simulink model "test14"  (R2019b)
settings: Solver=VariableStepAuto  StartTime=0.0  StopTime=10.0  RelTol=1e-3
settings Model: Creator=maxim  LastModifiedBy=maxim

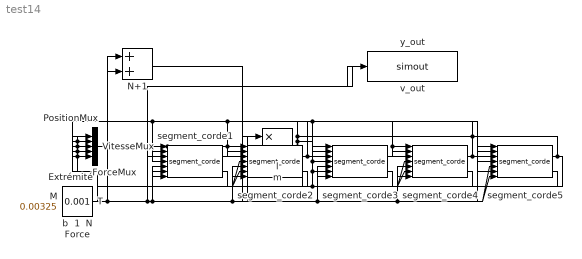
== system test14 ==
  1 : Constant
  Extrémité : Constant  Value=0
  Force : Constant  Value=0
  ForceMux : Mux  Inputs=5
  L : Constant  Value=0.443
  M : Constant  Value=0.00325
  N : Constant  Value=5
  N+1 : Sum
  PositionMux : Mux  Inputs=5
  T : Constant  Value=68.77
  VitesseMux : Mux  Inputs=5
  b : Constant  Value=0.001
  l : Product  Inputs=*/
  m : Product  Inputs=*/
  segment_corde{1..5} (5 alike) : M-S-Function  FunctionName=segment_corde
  v_out : ToWorkspace  VariableName=simout  SaveFormat=Timeseries  SampleTime=-1
  y_out : ToWorkspace  VariableName=simout  SaveFormat=Timeseries  SampleTime=-1
  wires:
  N/1 -> N+1/1, m/2
  1/1 -> N+1/2
  L/1 -> l/1
  N+1/1 -> l/2
  M/1 -> m/1
  m/1 -> segment_corde2/4, segment_corde4/4, segment_corde3/4, segment_corde1/4, segment_corde5/4
  T/1 -> segment_corde4/5, segment_corde5/5, segment_corde3/5, segment_corde2/5, segment_corde1/5
  l/1 -> segment_corde2/6, segment_corde4/6, segment_corde3/6, segment_corde5/6, segment_corde1/6
  b/1 -> segment_corde4/7, segment_corde5/7, segment_corde3/7, segment_corde2/7, segment_corde1/7
  segment_corde1/1 -> segment_corde2/1, PositionMux/1
  segment_corde2/1 -> segment_corde1/2, PositionMux/2, segment_corde3/1
  segment_corde3/1 -> segment_corde2/2, PositionMux/3, segment_corde4/1
  segment_corde4/1 -> segment_corde3/2, PositionMux/4, segment_corde5/1
  segment_corde5/1 -> segment_corde4/2, PositionMux/5
  Extrémité/1 -> segment_corde1/1, segment_corde5/2
  Force/1 -> ForceMux/1, ForceMux/2, ForceMux/3, ForceMux/4, ForceMux/5
  ForceMux/1 -> segment_corde2/3, segment_corde4/3, segment_corde3/3, segment_corde5/3, segment_corde1/3
  segment_corde1/2 -> VitesseMux/1
  segment_corde2/2 -> VitesseMux/2
  segment_corde3/2 -> VitesseMux/3
  segment_corde4/2 -> VitesseMux/4
  segment_corde5/2 -> VitesseMux/5
  PositionMux/1 -> y_out/1
  VitesseMux/1 -> v_out/1
